simulink model "P3cf"  (R2019b)
settings: Solver=FixedStepAuto  StartTime=0.0  StopTime=10.0  RelTol=1e-3  EnableMultiTasking=on
undefined symbols (not defined in the file): t_sim
libraries: legoev3lib x3, simulink x1
settings Model: ExtModeTrigDuration=2  Creator=alumnopr18  LastModifiedBy=alumnopr18
settings SolverCC: PositivePriorityOrder=on
settings OptimizationCC: EnhancedBackFolding=on  PassReuseOutputArgsAs=Individual arguments  ZeroExternalMemoryAtStartup=off  ZeroInternalMemoryAtStartup=off  MaxStackSize=64  OptimizeBlockOrder=speed  DifferentSizesBufferReuse=on  OptimizationCustomize=off  EfficientTunableParamExpr=on
settings DebuggingCC: ParameterTunabilityLossMsg=error
settings HardwareCC: ProdBitPerPointer=32  ProdBitPerSizeT=32  ProdBitPerPtrDiffT=32  ProdLargestAtomicInteger=Long  ProdWordSize=32  ProdHWDeviceType=ARM Compatible->ARM 9
settings SFSimCC: MATLABDynamicMemAlloc=off
settings RTWCC: SystemTargetFile=ert.tlc  HardwareBoard=LEGO MINDSTORMS EV3  TLCOptions="-aInlineSetEventsForThisBaseRateFcn=TLC_FALSE -aSuppressMultiTaskScheduler=TLC_FALSE  -aRateBasedStepFcn=0"  TemplateMakefile=ert_default_tmf  GenerateReport=on  Toolchain=Sourcery G++ Lite v2009q3  IncludeHyperlinkInReport=on  LaunchReport=on  GenerateTraceInfo=on  GenerateTraceReport=on  GenerateTraceReportSl=on  GenerateTraceReportSf=on  GenerateTraceReportEml=on
settings CodeAppCC: ForceParamTrailComments=on  IgnoreCustomStorageClasses=off  OperatorAnnotations=on  SimulinkDataObjDesc=on  SFDataObjDesc=on  InsertBlockDesc=on
settings ERTTargetCC: SupportContinuousTime=on  SupportVariableSizeSignals=on

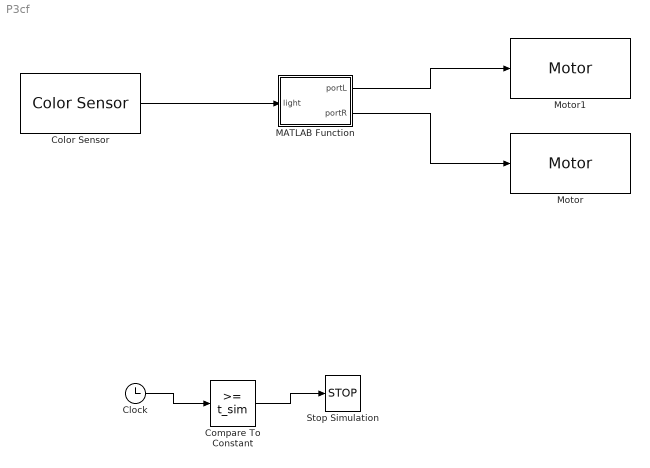
== system P3cf ==
  Clock : Clock
  Color Sensor : legoev3lib/Color Sensor  portNumber=4  mode=Reflected light intensity  sampleTime=0.1
      settings: SourceProductName=Simulink Support Package for LEGO MINDSTORMS EV3 Hardware  SourceProductBaseCode=LEGOEV3
  Compare To Constant : simulink/Logic and Bit Operations/Compare To Constant  relop=>=  const=t_sim  OutDataTypeStr=boolean
  MATLAB Function : MATLAB Function  TreatAsAtomicUnit=on
  Motor : legoev3lib/Motor  sportNumber=B  sstopAction=Brake
  Motor1 : legoev3lib/Motor  sportNumber=C  sstopAction=Brake
  Stop Simulation : Stop
  wires:
  Compare To Constant/1 -> Stop Simulation/1
  Clock/1 -> Compare To Constant/1
  Color Sensor/1 -> MATLAB Function/1(light)
  MATLAB Function/2(portR) -> Motor/1
  MATLAB Function/1(portL) -> Motor1/1

== matlab function P3cf/MATLAB Function ==
  data: light input; portL output; portR output
function [portL,portR] = fcn(light)
%Constantes
kp = 0.75;
ki = 0.02;
kd= 0.08;
windup = 30;
BLANCO = 70;
NEGRO = 35;
blanco = 90;
negro = 9;
%Persistent ya que en cada llamada se tiene que guardar la ultima
persistent lasterror 
persistent eintegral;
%Intervalo de muestreo
dt = 0.1;
%Inicialización de variables persistentes en la primera iteración
if(isempty(lasterror) || isempty(eintegral))
    lasterror = 0;
    eintegral = 0;
end
%Casteo a double de light
lectura = double(light);

%Normalización de la lectura del sensor
lecturarecta = (lectura*(BLANCO-NEGRO)/(blanco-negro))+ ((-negro*(BLANCO-NEGRO)) + (NEGRO*(blanco-negro)))/(blanco-negro);
%Calculo del error
error = lecturarecta - ((BLANCO+NEGRO)/2);


eintegral = eintegral + error*dt;
ederivada = (error - lasterror)/dt;

%Calculo de los componentes PID
proporcional = kp * error;
accionintegral = ki * eintegral;
accionder = kd * ederivada;
%PID total
u = proporcional + accionintegral + accionder;
%Uso del WINDUP para evitar el efecto windup
if (u > windup)
    u = u - accionintegral;
    eintegral = eintegral - error;
end
%Calculo de la potencia enviada a cada motor con la constante indicada
portL = 15 - u;
portR = 15 + u;

%Saturación
if(portL > 60)
    portL = 60;
end
if(portL < -60)
    portL = -60;
end
if(portR > 60)
    portR = 60;
end
if(portR < -60)
    portR = -60;
end

lasterror = error;
